simulink model "Battery_model_driving_cycle"  (R2019b)
settings: Solver=VariableStepAuto  StartTime=0.0  StopTime=10  RelTol=1e-3
undefined symbols (not defined in the file): A_frontal, air_density, Cn, Crate, Crate_fast, Cth, cv, fv, g, Gair, Gliquid, kt, m, Ob, Pn, Q_init, Rs1, rw, SOC_in, Temperature_BP, Tn, Vn
libraries: powerlib x27, simulink x10, drivingcycle_lib x2, powerlib_meascontrol x1
settings Model: Creator=Checco  LastModifiedBy=secch
settings SolverCC: ZeroCrossAlgorithm=Adaptive
settings DebuggingCC: IgnoredZcDiagnostic=none  ArithmeticOperatorsInVariantConditions=warning
settings SFSimCC: CustomCodeUndefinedFunction=UseInterfaceOnly

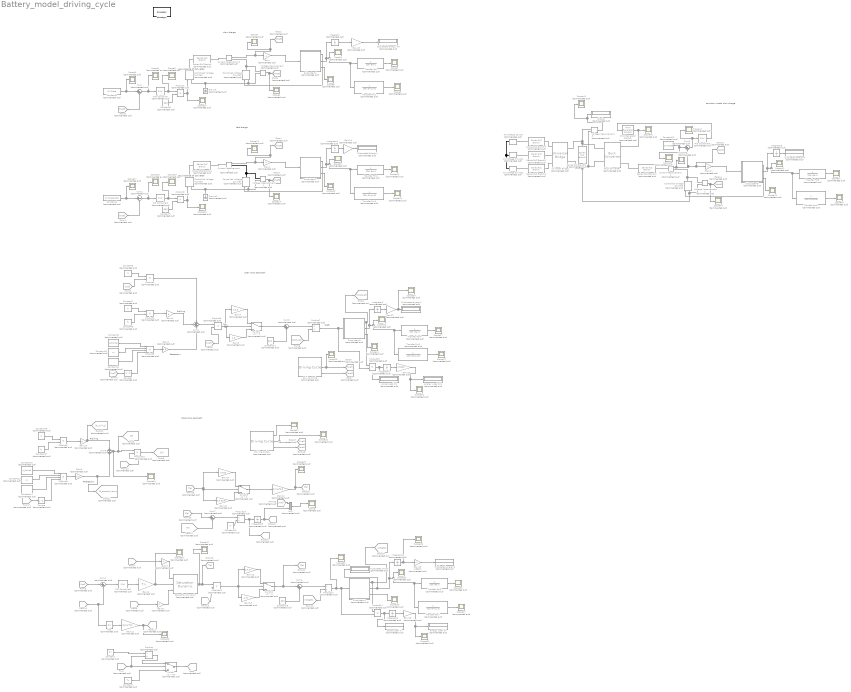
== system Battery_model_driving_cycle ==
  note: slow charge
  note: fast charge
  note: close loop approach
  note: open loop approach
  note: Ibatt
  note: Pm _
  note: Rrolling
  note: Raereodyn
  note: equivalence of converter
  note: equivalence of converter
  note: Rrolling
  note: Raereodyn
  note: complex model slow charge
  AC Voltage Source : powerlib/Electrical Sources/AC Voltage Source  Commented=on  Amplitude=230*sqrt(3)  Phase=0  Frequency=50  SampleTime=0  Measurements=None  BusType=swing  Pref=10e3  Qref=0  Qmin=-inf  Qmax=+inf
      settings: SourceProductName=Simscape Electrical
  AC Voltage Source1 : powerlib/Electrical Sources/AC Voltage Source  Commented=on  Amplitude=230*sqrt(3)  Phase=-120  Frequency=50  SampleTime=0  Measurements=None  BusType=swing  Pref=10e3  Qref=0  Qmin=-inf  Qmax=+inf
      settings: SourceProductName=Simscape Electrical
  AC Voltage Source2 : powerlib/Electrical Sources/AC Voltage Source  Commented=on  Amplitude=230*sqrt(3)  Phase=-240  Frequency=50  SampleTime=0  Measurements=None  BusType=swing  Pref=10e3  Qref=0  Qmin=-inf  Qmax=+inf
      settings: SourceProductName=Simscape Electrical
  Abs : Abs  Commented=on
  Buck Converter : powerlib/Power Electronics/Buck Converter  Commented=on  ModelType=Switching devices  Ron=1e-3  Rs=1e6  Cs=inf  Vforward=[0,0]  Ron_Diode=1e-3  Rs_Diode=1e6  Cs_Diode=inf  Vf_Diode=1e-3  Rs_CurrentSource=inf
      settings: SourceProductName=Simscape Electrical  SourceProductBaseCode=PS
  Constant : Constant  Commented=on  Value=Pn
  Constant1 : Constant  Commented=on  Value=Tn
  Constant10 : Constant  Commented=on  Value=cv
  Constant11 : Constant  Commented=on  Value=air_density
  Constant12 : Constant  Commented=on  Value=800
  Constant13 : Constant  Commented=on  Value=cv
  Constant14 : Constant  Commented=on  Value=air_density
  Constant{6..7,15,19} (4 alike) : Constant  Commented=on  Value=m
  Constant16 : Constant  Commented=on  Value=A_frontal
  Constant17 : Constant  Commented=on  Value=fv
  Constant18 : Constant  Commented=on  Value=800
  Constant2 : Constant  Commented=on  Value=Cn*Crate  SampleTime=-1
  Constant20 : Constant  Commented=on  Value=Cn*Crate  SampleTime=-1
  Constant3 : Constant  Commented=on  Value=560
  Constant4 : Constant  Commented=on  Value=Cn*Crate_fast  SampleTime=-1
  Constant5 : Constant  Commented=on  Value=560
  Constant8 : Constant  Commented=on  Value=A_frontal
  Constant9 : Constant  Commented=on  Value=fv
  Controlled Voltage Source1 : powerlib/Electrical Sources/Controlled Voltage Source  Commented=on  Initialize=off  Source_Type=DC  Amplitude=0.2*Cn  Phase=0  Frequency=0  Measurements=None
      settings: SourceProductName=Simscape Electrical
  Controlled Voltage Source2 : powerlib/Electrical Sources/Controlled Voltage Source  Commented=on  Initialize=off  Source_Type=DC  Amplitude=0  Phase=0  Frequency=0  Measurements=None
      settings: SourceProductName=Simscape Electrical
  Controlled Voltage Source3 : powerlib/Electrical Sources/Controlled Voltage Source  Commented=on  Initialize=off  Source_Type=DC  Amplitude=0.2*Cn  Phase=0  Frequency=0  Measurements=None
      settings: SourceProductName=Simscape Electrical
  Controlled Voltage Source4 : powerlib/Electrical Sources/Controlled Voltage Source  Commented=on  Initialize=off  Source_Type=DC  Amplitude=0  Phase=0  Frequency=0  Measurements=None
      settings: SourceProductName=Simscape Electrical
  Controlled Voltage Source6 : powerlib/Electrical Sources/Controlled Voltage Source  Commented=on  Initialize=off  Source_Type=DC  Amplitude=0  Phase=0  Frequency=0  Measurements=None
      settings: SourceProductName=Simscape Electrical
  Current Measurement : powerlib/Measurements/Current Measurement  Commented=on  PhasorSimulation=off  OutputType=Complex  PSBequivalent=0
      settings: SourceProductName=Simscape Electrical
  Current Measurement1 : powerlib/Measurements/Current Measurement  Commented=on  PhasorSimulation=off  OutputType=Complex  PSBequivalent=0
      settings: SourceProductName=Simscape Electrical
  Current Measurement2 : powerlib/Measurements/Current Measurement  Commented=on  PhasorSimulation=off  OutputType=Complex  PSBequivalent=0
      settings: SourceProductName=Simscape Electrical
  Display : Display  Commented=on
  Dissipated energy Wh : Display  Commented=on
  Dissipated energy{1..4} (4 alike) : Display  Commented=on
  Dissipated power : Display  Commented=on
  Driving Cycle : drivingcycle_lib/Driving Cycle  Commented=on  CycleName=NEDC  CycleRepeatsForever=off
      settings: SourceProductName=Driving Cycle Blockset
  Driving Cycle1 : drivingcycle_lib/Driving Cycle  Commented=on  CycleName=NEDC  CycleRepeatsForever=off
      settings: SourceProductName=Driving Cycle Blockset
  From : From  Commented=on  GotoTag=Omega
  From1 : From  Commented=on  GotoTag=Ibatt
  From10 : From  Commented=on  GotoTag=Vmeas
  From11 : From  Commented=on  GotoTag=Vmeas
  From12 : From  Commented=on  GotoTag=Vmeas
  From13 : From  Commented=on  GotoTag=Omega
  From14 : From  Commented=on  GotoTag=Vbatt
  From15 : From  Commented=on  GotoTag=Te
  From16 : From  Commented=on  GotoTag=Fe
  From17 : From  Commented=on  GotoTag=Fr
  From{4..5,9,18} (4 alike) : From  Commented=on  GotoTag=Vref
  From2 : From  Commented=on  GotoTag=Ibatt
  From3 : From  Commented=on  GotoTag=aref
  From6 : From  Commented=on  GotoTag=Vbatt_ref
  From7 : From  Commented=on  GotoTag=Tmax
  From8 : From  Commented=on  GotoTag=Tmax
  Gain{,1,8,17} (4 alike) : Gain  Commented=on  Gain=-1
  Gain10 : Gain  Commented=on  Gain=g
  Gain11 : Gain  Commented=on  Gain=1/rw*kt
  Gain12 : Gain  Commented=on  Gain=1/0.97
  Gain13 : Gain  Commented=on  Gain=0.97
  Gain14 : Gain  Commented=on  Gain=0.825
  Gain15 : Gain  Commented=on  Gain=1/0.825
  Gain16 : Gain  Commented=on  Gain=1/rw*kt
  Gain{18..23} (6 alike) : Gain  Commented=on  Gain=1/3600
  Gain2 : Gain  Commented=on  Gain=0.5
  Gain3 : Gain  Commented=on  Gain=g
  Gain4 : Gain  Commented=on  Gain=1/0.8
  Gain5 : Gain  Commented=on  Gain=0.8
  Gain6 : Gain  Commented=on  Gain=Tn
  Gain7 : Gain  Commented=on
  Gain9 : Gain  Commented=on  Gain=0.5
  Goto : Goto  Commented=on  GotoTag=Tmax
  Goto{1,3,14,19} (4 alike) : Goto  Commented=on  GotoTag=Vbatt
  Goto10 : Goto  Commented=on  GotoTag=R_rolling
  Goto11 : Goto  Commented=on  GotoTag=R_aereodynamic
  Goto12 : Goto  Commented=on  GotoTag=Omega
  Goto13 : Goto  Commented=on  GotoTag=Te
  Goto15 : Goto  Commented=on  GotoTag=Fe
  Goto16 : Goto  Commented=on  GotoTag=Vmeas
  Goto17 : Goto  Commented=on  GotoTag=Vref
  Goto18 : Goto  Commented=on  GotoTag=aref
  Goto2 : Goto  Commented=on  GotoTag=Ibatt
  Goto20 : Goto  Commented=on  GotoTag=ameas
  Goto21 : Goto  Commented=on  GotoTag=Pe
  Goto22 : Goto  Commented=on  GotoTag=Ibatt
  Goto4 : Goto  Commented=on  GotoTag=Ibatt
  Goto5 : Goto  Commented=on  GotoTag=Vbatt_ref
  Goto6 : Goto  Commented=on  GotoTag=Vref
  Goto7 : Goto  Commented=on  GotoTag=aref
  Goto8 : Goto  Commented=on  GotoTag=Fr
  Goto9 : Goto  Commented=on  GotoTag=Pr
  Ground : powerlib/Elements/Ground  Commented=on  LConnTagsString=a
      settings: SourceProductName=Simscape Electrical
  Ground1 : powerlib/Elements/Ground  Commented=on  LConnTagsString=a
      settings: SourceProductName=Simscape Electrical
  Integrator{,1..7} (8 alike) : Integrator  Commented=on
  Mux : Mux  Commented=on  Inputs=2
  PID Controller : simulink/Continuous/PID Controller  Commented=on  Controller=PI  Form=Parallel  TimeDomain=Continuous-time  SampleTime=-1  IntegratorMethod=Forward Euler  FilterMethod=Forward Euler  ControllerParametersSource=internal  P=0.01  I=1  D=0  UseFilter=on  N=100  TunerSelectOption=Transfer Function Based (PID Tuner App)  InitialConditionSource=internal  InitialConditionForIntegrator=370/560  InitialConditionForFilter=0  DifferentiatorICPrevScaledInput=0  ExternalReset=none  TrackingMode=off  Kt=1  LimitOutput=on  UpperSaturationLimit=1  LowerSaturationLimit=0  LinearizeAsGain=on  AntiWindupMode=none  Kb=1  POutMin=[]  POutMax=[]  IOutMin=[]  IOutMax=[]  DOutMin=[]  DOutMax=[]  NOutMin=[]  NOutMax=[]  SumOutMin=[]  SumOutMax=[]  SaturationOutMin=[]  SaturationOutMax=[]  PParamMin=[]  PParamMax=[]  IParamMin=[]  IParamMax=[]  DParamMin=[]  DParamMax=[]  NParamMin=[]  NParamMax=[]  KbParamMin=[]  KbParamMax=[]  KtParamMin=[]  KtParamMax=[]  KbOutMin=[]  KbOutMax=[]  KtOutMin=[]  KtOutMax=[]  IntegratorOutMin=[]  IntegratorOutMax=[]  FilterOutMin=[]  FilterOutMax=[]  SumI1OutMin=[]  SumI1OutMax=[]  SumI2OutMin=[]  SumI2OutMax=[]  SumI3OutMin=[]  SumI3OutMax=[]  SumI4OutMin=[]  SumI4OutMax=[]  SumDOutMin=[]  SumDOutMax=[]  DifferentiatorOutMin=[]  DifferentiatorOutMax=[]  FilterDiffOutCoefMin=[]  FilterDiffOutCoefMax=[]  ReciprocalOutMin=[]  ReciprocalOutMax=[]  SumDenOutMin=[]  SumDenOutMax=[]  SumNumOutMin=[]  SumNumOutMax=[]  DivideOutMin=[]  DivideOutMax=[]  IntegratorContinuousStateAttributes=''  IntegratorStateMustResolveToSignalObject=off  IntegratorRTWStateStorageClass=Auto  FilterContinuousStateAttributes=''  FilterStateMustResolveToSignalObject=off  FilterRTWStateStorageClass=Auto  ParallelPVariant=InternalParameters  IdealPVariant=Disabled  IVariant=InternalParameters  DVariant=Disabled  IntegratorVariant=Continuous  SatVariant=Enabled  AWVariant=Passthrough  PCopyVariant=Disabled  TRVariant=Disabled  FdbkBlocksVariant=Forward  IdealPFdbkVariant=Disabled  SatFdbkVariant=Disabled  DerivativeFilterVariant=Disabled  NVariant=Disabled  NCopyVariant=Disabled_SignalSpec  FilterICVariant=Disabled  IntegratorICVariant=InternalICs  ExternalResetVariant=Disabled  TRSumVariant=Passthrough  SumFdbkVariant=Disabled  SumVariant=Sum_PI
  PID Controller1 : simulink/Continuous/PID Controller  Commented=on  Controller=PI  Form=Parallel  TimeDomain=Continuous-time  SampleTime=-1  IntegratorMethod=Forward Euler  FilterMethod=Forward Euler  ControllerParametersSource=internal  P=0.01  I=1  D=0  UseFilter=on  N=100  TunerSelectOption=Transfer Function Based (PID Tuner App)  InitialConditionSource=internal  InitialConditionForIntegrator=370/560  InitialConditionForFilter=0  DifferentiatorICPrevScaledInput=0  ExternalReset=none  TrackingMode=off  Kt=1  LimitOutput=on  UpperSaturationLimit=1  LowerSaturationLimit=0  LinearizeAsGain=on  AntiWindupMode=none  Kb=1  POutMin=[]  POutMax=[]  IOutMin=[]  IOutMax=[]  DOutMin=[]  DOutMax=[]  NOutMin=[]  NOutMax=[]  SumOutMin=[]  SumOutMax=[]  SaturationOutMin=[]  SaturationOutMax=[]  PParamMin=[]  PParamMax=[]  IParamMin=[]  IParamMax=[]  DParamMin=[]  DParamMax=[]  NParamMin=[]  NParamMax=[]  KbParamMin=[]  KbParamMax=[]  KtParamMin=[]  KtParamMax=[]  KbOutMin=[]  KbOutMax=[]  KtOutMin=[]  KtOutMax=[]  IntegratorOutMin=[]  IntegratorOutMax=[]  FilterOutMin=[]  FilterOutMax=[]  SumI1OutMin=[]  SumI1OutMax=[]  SumI2OutMin=[]  SumI2OutMax=[]  SumI3OutMin=[]  SumI3OutMax=[]  SumI4OutMin=[]  SumI4OutMax=[]  SumDOutMin=[]  SumDOutMax=[]  DifferentiatorOutMin=[]  DifferentiatorOutMax=[]  FilterDiffOutCoefMin=[]  FilterDiffOutCoefMax=[]  ReciprocalOutMin=[]  ReciprocalOutMax=[]  SumDenOutMin=[]  SumDenOutMax=[]  SumNumOutMin=[]  SumNumOutMax=[]  DivideOutMin=[]  DivideOutMax=[]  IntegratorContinuousStateAttributes=''  IntegratorStateMustResolveToSignalObject=off  IntegratorRTWStateStorageClass=Auto  FilterContinuousStateAttributes=''  FilterStateMustResolveToSignalObject=off  FilterRTWStateStorageClass=Auto  ParallelPVariant=InternalParameters  IdealPVariant=Disabled  IVariant=InternalParameters  DVariant=Disabled  IntegratorVariant=Continuous  SatVariant=Enabled  AWVariant=Passthrough  PCopyVariant=Disabled  TRVariant=Disabled  FdbkBlocksVariant=Forward  IdealPFdbkVariant=Disabled  SatFdbkVariant=Disabled  DerivativeFilterVariant=Disabled  NVariant=Disabled  NCopyVariant=Disabled_SignalSpec  FilterICVariant=Disabled  IntegratorICVariant=InternalICs  ExternalResetVariant=Disabled  TRSumVariant=Passthrough  SumFdbkVariant=Disabled  SumVariant=Sum_PI
  PID Controller2 : simulink/Continuous/PID Controller  Commented=on  Controller=PI  Form=Parallel  TimeDomain=Continuous-time  SampleTime=-1  IntegratorMethod=Forward Euler  FilterMethod=Forward Euler  ControllerParametersSource=internal  P=1  I=100  D=0  UseFilter=on  N=100  TunerSelectOption=Transfer Function Based (PID Tuner App)  InitialConditionSource=internal  InitialConditionForIntegrator=0  InitialConditionForFilter=0  DifferentiatorICPrevScaledInput=0  ExternalReset=none  TrackingMode=off  Kt=1  LimitOutput=on  UpperSaturationLimit=1  LowerSaturationLimit=-1  LinearizeAsGain=on  AntiWindupMode=none  Kb=1  POutMin=[]  POutMax=[]  IOutMin=[]  IOutMax=[]  DOutMin=[]  DOutMax=[]  NOutMin=[]  NOutMax=[]  SumOutMin=[]  SumOutMax=[]  SaturationOutMin=[]  SaturationOutMax=[]  PParamMin=[]  PParamMax=[]  IParamMin=[]  IParamMax=[]  DParamMin=[]  DParamMax=[]  NParamMin=[]  NParamMax=[]  KbParamMin=[]  KbParamMax=[]  KtParamMin=[]  KtParamMax=[]  KbOutMin=[]  KbOutMax=[]  KtOutMin=[]  KtOutMax=[]  IntegratorOutMin=[]  IntegratorOutMax=[]  FilterOutMin=[]  FilterOutMax=[]  SumI1OutMin=[]  SumI1OutMax=[]  SumI2OutMin=[]  SumI2OutMax=[]  SumI3OutMin=[]  SumI3OutMax=[]  SumI4OutMin=[]  SumI4OutMax=[]  SumDOutMin=[]  SumDOutMax=[]  DifferentiatorOutMin=[]  DifferentiatorOutMax=[]  FilterDiffOutCoefMin=[]  FilterDiffOutCoefMax=[]  ReciprocalOutMin=[]  ReciprocalOutMax=[]  SumDenOutMin=[]  SumDenOutMax=[]  SumNumOutMin=[]  SumNumOutMax=[]  DivideOutMin=[]  DivideOutMax=[]  IntegratorContinuousStateAttributes=''  IntegratorStateMustResolveToSignalObject=off  IntegratorRTWStateStorageClass=Auto  FilterContinuousStateAttributes=''  FilterStateMustResolveToSignalObject=off  FilterRTWStateStorageClass=Auto  ParallelPVariant=InternalParameters  IdealPVariant=Disabled  IVariant=InternalParameters  DVariant=Disabled  IntegratorVariant=Continuous  SatVariant=Enabled  AWVariant=Passthrough  PCopyVariant=Disabled  TRVariant=Disabled  FdbkBlocksVariant=Forward  IdealPFdbkVariant=Disabled  SatFdbkVariant=Disabled  DerivativeFilterVariant=Disabled  NVariant=Disabled  NCopyVariant=Disabled_SignalSpec  FilterICVariant=Disabled  IntegratorICVariant=InternalICs  ExternalResetVariant=Disabled  TRSumVariant=Passthrough  SumFdbkVariant=Disabled  SumVariant=Sum_PI
  PID Controller3 : simulink/Continuous/PID Controller  Commented=on  Controller=PI  Form=Parallel  TimeDomain=Continuous-time  SampleTime=-1  IntegratorMethod=Forward Euler  FilterMethod=Forward Euler  ControllerParametersSource=internal  P=0.01  I=1  D=0  UseFilter=on  N=100  TunerSelectOption=Transfer Function Based (PID Tuner App)  InitialConditionSource=internal  InitialConditionForIntegrator=Vn/560  InitialConditionForFilter=0  DifferentiatorICPrevScaledInput=0  ExternalReset=none  TrackingMode=off  Kt=1  LimitOutput=on  UpperSaturationLimit=1  LowerSaturationLimit=0  LinearizeAsGain=on  AntiWindupMode=none  Kb=1  POutMin=[]  POutMax=[]  IOutMin=[]  IOutMax=[]  DOutMin=[]  DOutMax=[]  NOutMin=[]  NOutMax=[]  SumOutMin=[]  SumOutMax=[]  SaturationOutMin=[]  SaturationOutMax=[]  PParamMin=[]  PParamMax=[]  IParamMin=[]  IParamMax=[]  DParamMin=[]  DParamMax=[]  NParamMin=[]  NParamMax=[]  KbParamMin=[]  KbParamMax=[]  KtParamMin=[]  KtParamMax=[]  KbOutMin=[]  KbOutMax=[]  KtOutMin=[]  KtOutMax=[]  IntegratorOutMin=[]  IntegratorOutMax=[]  FilterOutMin=[]  FilterOutMax=[]  SumI1OutMin=[]  SumI1OutMax=[]  SumI2OutMin=[]  SumI2OutMax=[]  SumI3OutMin=[]  SumI3OutMax=[]  SumI4OutMin=[]  SumI4OutMax=[]  SumDOutMin=[]  SumDOutMax=[]  DifferentiatorOutMin=[]  DifferentiatorOutMax=[]  FilterDiffOutCoefMin=[]  FilterDiffOutCoefMax=[]  ReciprocalOutMin=[]  ReciprocalOutMax=[]  SumDenOutMin=[]  SumDenOutMax=[]  SumNumOutMin=[]  SumNumOutMax=[]  DivideOutMin=[]  DivideOutMax=[]  IntegratorContinuousStateAttributes=''  IntegratorStateMustResolveToSignalObject=off  IntegratorRTWStateStorageClass=Auto  FilterContinuousStateAttributes=''  FilterStateMustResolveToSignalObject=off  FilterRTWStateStorageClass=Auto  ParallelPVariant=InternalParameters  IdealPVariant=Disabled  IVariant=InternalParameters  DVariant=Disabled  IntegratorVariant=Continuous  SatVariant=Enabled  AWVariant=Passthrough  PCopyVariant=Disabled  TRVariant=Disabled  FdbkBlocksVariant=Forward  IdealPFdbkVariant=Disabled  SatFdbkVariant=Disabled  DerivativeFilterVariant=Disabled  NVariant=Disabled  NCopyVariant=Disabled_SignalSpec  FilterICVariant=Disabled  IntegratorICVariant=InternalICs  ExternalResetVariant=Disabled  TRSumVariant=Passthrough  SumFdbkVariant=Disabled  SumVariant=Sum_PI
  PWM Generator (DC-DC) : powerlib_meascontrol/Pulse & Signal Generators/PWM Generator (DC-DC)  Commented=on  Fsw=5000  Ts=0
      settings: SourceProductName=Simscape Electrical
  Product{,7,12..13} (4 alike) : Product  Commented=on  Inputs=*/
  Product{1..4,6,8,10..11} (8 alike) : Product  Commented=on
  Product14 : Product  Commented=on  Inputs=**
  Product15 : Product  Commented=on  Inputs=**
  Product5 : Product  Commented=on  Inputs=4
  Product9 : Product  Commented=on  Inputs=4
  Saturation Dynamic : simulink/Discontinuities/Saturation Dynamic  Commented=on  OutMin=[]  OutMax=[]  OutDataTypeStr=Inherit: Same as second input  OutDataType=fixdt(1, 16)  OutScaling=2^-10  DoSatur=off
  Scope{,1..51} (52 alike) : Scope  Commented=on
  Series RLC Branch : powerlib/Elements/Series RLC Branch  Commented=on  LConnTagsString=__new0  RConnTagsString=__new0  BranchType=RL  Resistance=0.0001  Inductance=0.01  SetiL0=off  InitialCurrent=0  Capacitance=1e-6  Setx0=off  InitialVoltage=0  Measurements=None
      settings: SourceProductName=Simscape Electrical
  Series RLC Branch1 : powerlib/Elements/Series RLC Branch  Commented=on  LConnTagsString=__new0  RConnTagsString=__new0  BranchType=RL  Resistance=0.0001  Inductance=0.01  SetiL0=off  InitialCurrent=0  Capacitance=1e-6  Setx0=off  InitialVoltage=0  Measurements=None
      settings: SourceProductName=Simscape Electrical
  Series RLC Branch2 : powerlib/Elements/Series RLC Branch  Commented=on  LConnTagsString=__new0  RConnTagsString=__new0  BranchType=RL  Resistance=3  Inductance=1e-3  SetiL0=off  InitialCurrent=0  Capacitance=1e-6  Setx0=off  InitialVoltage=0  Measurements=None
      settings: SourceProductName=Simscape Electrical
  Series RLC Branch3 : powerlib/Elements/Series RLC Branch  Commented=on  LConnTagsString=__new0  RConnTagsString=__new0  BranchType=RL  Resistance=3  Inductance=1e-3  SetiL0=off  InitialCurrent=0  Capacitance=1e-6  Setx0=off  InitialVoltage=0  Measurements=None
      settings: SourceProductName=Simscape Electrical
  Series RLC Branch4 : powerlib/Elements/Series RLC Branch  Commented=on  LConnTagsString=__new0  RConnTagsString=__new0  BranchType=RL  Resistance=3  Inductance=1e-3  SetiL0=off  InitialCurrent=0  Capacitance=1e-6  Setx0=off  InitialVoltage=0  Measurements=None
      settings: SourceProductName=Simscape Electrical
  Series RLC Branch6 : powerlib/Elements/Series RLC Branch  Commented=on  LConnTagsString=__new0  RConnTagsString=__new0  BranchType=C  Resistance=0.0001  Inductance=0.01  SetiL0=off  InitialCurrent=0  Capacitance=600e-6  Setx0=off  InitialVoltage=0  Measurements=None
      settings: SourceProductName=Simscape Electrical
  Series RLC Branch7 : powerlib/Elements/Series RLC Branch  Commented=on  LConnTagsString=__new0  RConnTagsString=__new0  BranchType=RL  Resistance=0.0001  Inductance=0.01  SetiL0=off  InitialCurrent=0  Capacitance=1e-6  Setx0=off  InitialVoltage=0  Measurements=None
      settings: SourceProductName=Simscape Electrical
  Square : Math  Commented=on  Operator=square  SignedPower=off  SaturateOnIntegerOverflow=on
  Square1 : Math  Commented=on  Operator=square  SignedPower=off  SaturateOnIntegerOverflow=on
  Subsystem1 : Subsystem  Commented=on  mask{Em=|, R0=0.0036, SOC_BP=|, BattCap=31, SOC_ini=20, Ns=100, Np=3}
      mask Em=|
      | [3;
      | 3.5 ;
      | 3.67 ;
      | 3.7 ;
      | 3.71 ;
      | 3.72 ;
      | 3.73 ;
      | 3.74 ;
      | 3.75 ;
      | 3.84;
      | 4.2]
      mask SOC_BP=|
      | [0
      | 0.1
      | 0.2
      | 0.3
      | 0.4
      | 0.5
      | 0.6
      | 0.7
      | 0.8
      | 0.9
      | 1]
      mask prompts: Em "Open circuit voltage table data, Em [V]:"; R0 "Series resistance R0 [Ohm]:"; SOC_BP "State of charge breakpoints, SOC_BP []"; BattCap "Battery capacity, BattCap [Ah]"; SOC_ini "SOC ini [%]"; Ns "Num Series"; Np "Num Parallel"
      mask DialogControl Control3 Prompt: Single Module Data
      mask DialogControl Control2 Prompt: Connections
  Subsystem2 : Subsystem  Commented=on  mask{Em=|, R0=0.0036, SOC_BP=|, BattCap=31, SOC_ini=20, Ns=100, Np=3}
      mask Em=|
      | [3;
      | 3.5 ;
      | 3.67 ;
      | 3.7 ;
      | 3.71 ;
      | 3.72 ;
      | 3.73 ;
      | 3.74 ;
      | 3.75 ;
      | 3.84;
      | 4.2]
      mask SOC_BP=|
      | [0
      | 0.1
      | 0.2
      | 0.3
      | 0.4
      | 0.5
      | 0.6
      | 0.7
      | 0.8
      | 0.9
      | 1]
      mask prompts: Em "Open circuit voltage table data, Em [V]:"; R0 "Series resistance R0 [Ohm]:"; SOC_BP "State of charge breakpoints, SOC_BP []"; BattCap "Battery capacity, BattCap [Ah]"; SOC_ini "SOC ini [%]"; Ns "Num Series"; Np "Num Parallel"
      mask DialogControl Control3 Prompt: Single Module Data
      mask DialogControl Control2 Prompt: Connections
  Subsystem3 : Subsystem  Commented=on  mask{Em=|, R0=0.0036, SOC_BP=|, BattCap=31, SOC_ini=100, Ns=100, Np=3}
      mask Em=|
      | [3;
      | 3.5 ;
      | 3.67 ;
      | 3.7 ;
      | 3.71 ;
      | 3.72 ;
      | 3.73 ;
      | 3.74 ;
      | 3.75 ;
      | 3.84;
      | 4.2]
      mask SOC_BP=|
      | [0
      | 0.1
      | 0.2
      | 0.3
      | 0.4
      | 0.5
      | 0.6
      | 0.7
      | 0.8
      | 0.9
      | 1]
      mask prompts: Em "Open circuit voltage table data, Em [V]:"; R0 "Series resistance R0 [Ohm]:"; SOC_BP "State of charge breakpoints, SOC_BP []"; BattCap "Battery capacity, BattCap [Ah]"; SOC_ini "SOC ini [%]"; Ns "Num Series"; Np "Num Parallel"
      mask DialogControl Control3 Prompt: Single Module Data
      mask DialogControl Control2 Prompt: Connections
  Subsystem4 : Subsystem  Commented=on  mask{Em=|, R0=0.0036, SOC_BP=|, BattCap=31, SOC_ini=100, Ns=100, Np=3}
      mask Em=|
      | [3;
      | 3.5 ;
      | 3.67 ;
      | 3.7 ;
      | 3.71 ;
      | 3.72 ;
      | 3.73 ;
      | 3.74 ;
      | 3.75 ;
      | 3.84;
      | 4.2]
      mask SOC_BP=|
      | [0
      | 0.1
      | 0.2
      | 0.3
      | 0.4
      | 0.5
      | 0.6
      | 0.7
      | 0.8
      | 0.9
      | 1]
      mask prompts: Em "Open circuit voltage table data, Em [V]:"; R0 "Series resistance R0 [Ohm]:"; SOC_BP "State of charge breakpoints, SOC_BP []"; BattCap "Battery capacity, BattCap [Ah]"; SOC_ini "SOC ini [%]"; Ns "Num Series"; Np "Num Parallel"
      mask DialogControl Control3 Prompt: Single Module Data
      mask DialogControl Control2 Prompt: Connections
  Subsystem5 : Subsystem  Commented=on  mask{Em=|, R0=0.0036, SOC_BP=|, BattCap=31, SOC_ini=20, Ns=100, Np=3}
      mask Em=|
      | [3;
      | 3.5 ;
      | 3.67 ;
      | 3.7 ;
      | 3.71 ;
      | 3.72 ;
      | 3.73 ;
      | 3.74 ;
      | 3.75 ;
      | 3.84;
      | 4.2]
      mask SOC_BP=|
      | [0
      | 0.1
      | 0.2
      | 0.3
      | 0.4
      | 0.5
      | 0.6
      | 0.7
      | 0.8
      | 0.9
      | 1]
      mask prompts: Em "Open circuit voltage table data, Em [V]:"; R0 "Series resistance R0 [Ohm]:"; SOC_BP "State of charge breakpoints, SOC_BP []"; BattCap "Battery capacity, BattCap [Ah]"; SOC_ini "SOC ini [%]"; Ns "Num Series"; Np "Num Parallel"
      mask DialogControl Control3 Prompt: Single Module Data
      mask DialogControl Control2 Prompt: Connections
  Sum{,1,4,7..8} (5 alike) : Sum  Commented=on  Inputs=|+-
  Sum2 : Sum  Commented=on  Inputs=+++
  Sum3 : Sum  Commented=on  Inputs=|++
  Sum5 : Sum  Commented=on
  Sum6 : Sum  Commented=on  Inputs=|++
  Switch : Switch  Commented=on  Criteria=u2 > Threshold  Threshold=Ob
  Switch1 : Switch  Commented=on  Criteria=u2 > Threshold
  Switch2 : Switch  Commented=on  Criteria=u2 > Threshold
  Switch3 : Switch  Commented=on  Criteria=u2 > Threshold
  Transfer Fcn{,2,4,6,8} (5 alike) : TransferFcn  Commented=on  Denominator=[Cth Gair]
  Transfer Fcn{1,3,5,7,9} (5 alike) : TransferFcn  Commented=on  Denominator=[Cth Gliquid]
  Universal Bridge : powerlib/Power Electronics/Universal Bridge  Commented=on  Arms=3  SnubberResistance=1e5  SnubberCapacitance=inf  Device=Diodes  Ron=1e-3  Lon=0  ForwardVoltages="[  0  0  ]"  ForwardVoltage=0  GTOparameters=[ 10e-6 , 20e-6 ]  IGBTparameters=[ 1e-6 , 2e-6 ]  Measurements=None  Measurements_2=None  converterType=Rectifier
      settings: SourceProductName=Simscape Electrical
  Voltage Measurement{,1..3} (4 alike) : powerlib/Measurements/Voltage Measurement  Commented=on  PhasorSimulation=off  OutputType=Complex  PSBequivalent=0
      settings: SourceProductName=Simscape Electrical
  energy used wh : Display  Commented=on
  energy used wh1 : Display  Commented=on
  power used W : Display  Commented=on
  power used W1 : Display  Commented=on
  powergui : powerlib/powergui  Priority=1  SimulationMode=Continuous  SampleTime=50e-6  frequency=60  Iterations=50  frequencyindice=0  Pbase=100e6  ErrMax=1e-4  UnitsV=kV  UnitsW=MW  buscounter=0  FunctionMessages=off  echomessages=off  EnableUseOfTLC=off  CurrentSourceSwitches=off  DisableSnubberDevices=off  DisableRonSwitches=off  DisableVfSwitches=off  DisplayEquations=off  AutomaticDiscreteSolvers=off  SolverType=Tustin/Backward Euler (TBE)  Interpol=off  ExternalGateDelay=off  methode=off  Ts=100  x0status=blocks  SPID=on  SwTol=0  HookPort=off  NonlinearTolerance=1e-4  nMaxIteration=100  ContinueOnMaxIteration=off  RestoreLinks=warning  ResistiveCurrentMeasurement=off  Frange=[0:2:500]  Ylog=off  Xlog=on  ShowGrid=off  save=off  variable=ZData  structure=0  ZoomFFT=off  StartTime=0.0  cycles=1  DisplayStyle=1  fundamental=60  FreqAxis=off  MaxFrequency=1000  frequencyindicesteady=1  RmsSteady=1  display=off
      settings: SourceProductName=Simscape Electrical
  wires:
  From2/1 -> Sum/2
  Sum/1 -> Scope5/1, PID Controller/1
  PID Controller/1 -> Scope8/1, Product1/1
  Constant3/1 -> Product1/2
  Product1/1 -> Scope10/1, Controlled Voltage Source1/1
  Voltage Measurement/1 -> Scope4/1, Goto1/1
  Current Measurement/1 -> Goto2/1, Scope7/1, Gain/1
  Gain/1 -> Subsystem1/1(Ibatt)
  Subsystem1/2(Ploss) -> Scope1/1, Transfer Fcn1/1, Transfer Fcn/1, Integrator/1
  Integrator/1 -> Gain20/1
  Subsystem1/3(SOC) -> Scope9/1
  Transfer Fcn/1 -> Scope2/1
  Transfer Fcn1/1 -> Scope3/1
  Subsystem1/1(Vbatt) -> Controlled Voltage Source2/1
  Constant2/1 -> Scope6/1, Sum/1
  Constant4/1 -> Sum1/1, Scope17/1
  Subsystem2/1(Vbatt) -> Controlled Voltage Source4/1
  Transfer Fcn3/1 -> Scope14/1
  Transfer Fcn2/1 -> Scope13/1
  Subsystem2/3(SOC) -> Scope20/1
  Integrator1/1 -> Gain21/1
  Subsystem2/2(Ploss) -> Integrator1/1, Transfer Fcn2/1, Transfer Fcn3/1, Scope11/1
  Gain1/1 -> Subsystem2/1(Ibatt)
  Current Measurement1/1 -> Gain1/1, Scope18/1, Goto4/1
  Voltage Measurement1/1 -> Goto3/1, Scope15/1
  Product2/1 -> Controlled Voltage Source3/1, Scope12/1
  Constant5/1 -> Product2/2
  PID Controller1/1 -> Product2/1, Scope19/1
  Sum1/1 -> PID Controller1/1, Scope16/1
  From1/1 -> Sum1/2
  Constant6/1 -> Product3/1
  From3/1 -> Product3/2
  Constant9/1 -> Product4/2
  Constant7/1 -> Product4/1
  Constant8/1 -> Product5/1
  Constant10/1 -> Product5/2
  Constant11/1 -> Product5/3
  From4/1 -> Square1/1
  Product5/1 -> Gain2/1
  Product4/1 -> Gain3/1
  Product3/1 -> Sum2/1
  Gain3/1 -> Sum2/2
  Gain2/1 -> Sum2/3
  Sum2/1 -> Product6/1
  From5/1 -> Product6/2
  Product6/1 -> Gain4/1, Gain5/1, Switch1/2
  Gain5/1 -> Switch1/3
  Gain4/1 -> Switch1/1
  Switch1/1 -> Sum3/1
  Constant12/1 -> Sum3/2
  Sum3/1 -> Product7/1
  From6/1 -> Product7/2
  Subsystem3/2(Ploss) -> Integrator2/1, Scope21/1, Transfer Fcn5/1, Transfer Fcn4/1
  Subsystem3/3(SOC) -> Scope24/1
  Transfer Fcn4/1 -> Scope22/1
  Transfer Fcn5/1 -> Scope23/1
  Product7/1 -> Product15/2, Subsystem3/1(Ibatt)
  Integrator2/1 -> Gain22/1
  Subsystem3/1(Vbatt) -> Goto5/1, Product15/1
  PID Controller2/1 -> Gain6/1
  Gain6/1 -> Scope33/1, Saturation Dynamic/2
  Gain8/1 -> Saturation Dynamic/3
  Gain7/1 -> Saturation Dynamic/1
  From7/1 -> Gain7/1
  From8/1 -> Gain8/1
  From9/1 -> Sum4/1
  Sum4/1 -> PID Controller2/1
  From10/1 -> Abs/1, Sum4/2
  Driving Cycle/2 -> Scope29/1, Goto6/1
  Driving Cycle/3 -> Goto7/1
  Product9/1 -> Gain9/1
  Constant14/1 -> Product9/3
  Gain9/1 -> Sum5/2, Goto11/1
  Constant16/1 -> Product9/1
  From11/1 -> Square/1
  Constant13/1 -> Product9/2
  Gain10/1 -> Sum5/1, Goto10/1
  Constant15/1 -> Product8/1
  Constant17/1 -> Product8/2
  Product8/1 -> Gain10/1
  Sum5/1 -> Scope34/1, Goto8/1, Product10/1
  From12/1 -> Product10/2
  Product10/1 -> Goto9/1
  Abs/1 -> Gain11/1
  Gain11/1 -> Scope39/1, Goto12/1
  Saturation Dynamic/1 -> Scope32/1, Goto13/1, Product11/1
  From13/1 -> Product11/2
  Product11/1 -> Gain12/1, Gain13/1, Switch2/2
  Constant18/1 -> Sum6/2
  Switch2/1 -> Goto21/1, Sum6/1
  Sum6/1 -> Product12/1
  From14/1 -> Product12/2
  Gain12/1 -> Switch2/1
  Gain13/1 -> Switch2/3
  Product/1 -> Switch/1
  Constant1/1 -> Switch/3
  Constant/1 -> Product/1
  From/1 -> Product/2, Switch/2
  Switch/1 -> Goto/1
  Gain15/1 -> Switch3/3
  Gain14/1 -> Switch3/1
  From15/1 -> Switch3/2, Gain15/1, Gain14/1
  Switch3/1 -> Gain16/1
  Gain16/1 -> Scope35/1, Goto15/1
  From16/1 -> Sum7/1
  From17/1 -> Sum7/2
  Sum7/1 -> Product13/1
  Constant19/1 -> Product13/2
  Product13/1 -> Goto20/1, Integrator3/1
  Integrator3/1 -> Mux/2, Goto16/1
  Driving Cycle1/3 -> Goto18/1
  Driving Cycle1/2 -> Scope31/1, Goto17/1
  Product12/1 -> Scope38/1, Product14/2, Subsystem4/1(Ibatt)
  Subsystem4/1(Vbatt) -> Product14/1, Goto19/1
  Integrator4/1 -> Scope36/1, Gain19/1
  Transfer Fcn7/1 -> Scope27/1
  Transfer Fcn6/1 -> Scope26/1
  Subsystem4/3(SOC) -> Scope28/1
  Subsystem4/2(Ploss) -> Dissipated power/1, Transfer Fcn6/1, Transfer Fcn7/1, Scope25/1, Integrator4/1
  Mux/1 -> Scope/1
  From18/1 -> Mux/1
  Driving Cycle1/1 -> Scope37/1
  Subsystem5/2(Ploss) -> Scope40/1, Transfer Fcn9/1, Transfer Fcn8/1, Integrator5/1
  Transfer Fcn9/1 -> Scope43/1
  Subsystem5/3(SOC) -> Scope49/1
  Gain17/1 -> Subsystem5/1(Ibatt)
  Current Measurement2/1 -> Scope45/1, Goto22/1, Gain17/1, Sum8/2
  Subsystem5/1(Vbatt) -> Controlled Voltage Source6/1
  Voltage Measurement2/1 -> Scope44/1, Goto14/1
  Transfer Fcn8/1 -> Scope42/1
  Integrator5/1 -> Dissipated energy4/1
  Constant20/1 -> Scope48/1, Sum8/1
  Sum8/1 -> Scope47/1, PID Controller3/1
  PID Controller3/1 -> PWM Generator (DC-DC)/1
  PWM Generator (DC-DC)/1 -> Buck Converter/1, Scope46/1
  Voltage Measurement3/1 -> Scope41/1, Display/1
  Product14/1 -> power used W/1, Integrator6/1
  Integrator6/1 -> Gain18/1
  Gain18/1 -> Scope50/1, energy used wh/1
  Gain19/1 -> Dissipated energy3/1
  Square/1 -> Product9/4
  Square1/1 -> Product5/4
  Gain20/1 -> Dissipated energy Wh/1
  Gain21/1 -> Dissipated energy1/1
  Gain22/1 -> Scope30/1, Dissipated energy2/1
  Gain23/1 -> energy used wh1/1, Scope51/1
  Integrator7/1 -> Gain23/1
  Product15/1 -> Integrator7/1, power used W1/1
  connections:
  Series RLC Branch/LConn1 -- Controlled Voltage Source1/RConn1
  Current Measurement/LConn1 -- Series RLC Branch/RConn1
  Controlled Voltage Source2/RConn1 -- Current Measurement/RConn1 -- Voltage Measurement/LConn1
  Controlled Voltage Source2/LConn1 -- Ground/LConn1 -- Controlled Voltage Source1/LConn1 -- Voltage Measurement/LConn2
  Current Measurement1/RConn1 -- Controlled Voltage Source4/RConn1 -- Voltage Measurement1/LConn1
  Voltage Measurement1/LConn2 -- Controlled Voltage Source4/LConn1 -- Controlled Voltage Source3/LConn1 -- Ground1/LConn1
  Current Measurement1/LConn1 -- Series RLC Branch1/RConn1
  Series RLC Branch1/LConn1 -- Controlled Voltage Source3/RConn1
  Voltage Measurement2/LConn1 -- Controlled Voltage Source6/RConn1 -- Current Measurement2/RConn1
  AC Voltage Source/RConn1 -- Series RLC Branch3/LConn1
  Series RLC Branch2/LConn1 -- AC Voltage Source1/RConn1
  Series RLC Branch4/LConn1 -- AC Voltage Source2/RConn1
  AC Voltage Source/LConn1 -- AC Voltage Source2/LConn1 -- AC Voltage Source1/LConn1
  Series RLC Branch2/RConn1 -- Universal Bridge/LConn2
  Universal Bridge/LConn1 -- Series RLC Branch3/RConn1
  Series RLC Branch4/RConn1 -- Universal Bridge/LConn3
  Series RLC Branch6/LConn1 -- Buck Converter/RConn1 -- Voltage Measurement3/LConn1 -- Universal Bridge/RConn1
  Series RLC Branch6/RConn1 -- Buck Converter/RConn2 -- Voltage Measurement3/LConn2 -- Voltage Measurement2/LConn2 -- Controlled Voltage Source6/LConn1 -- Universal Bridge/RConn2
  Series RLC Branch7/LConn1 -- Buck Converter/LConn1
  Current Measurement2/LConn1 -- Series RLC Branch7/RConn1

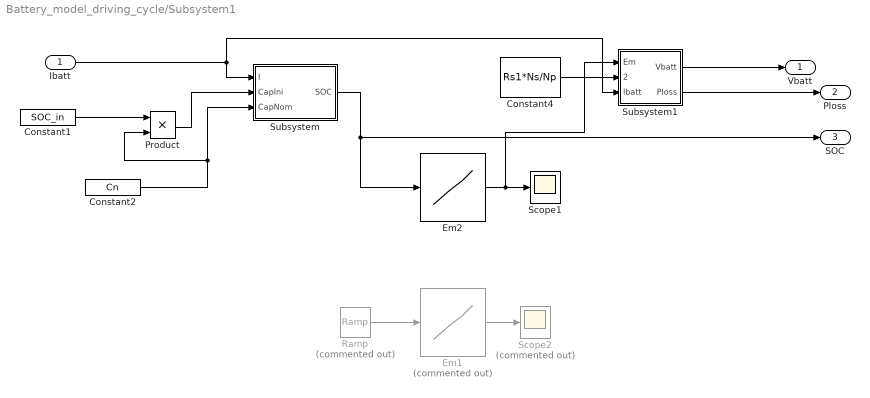
== system Battery_model_driving_cycle/Subsystem1 ==
  Ibatt : Inport
  Constant1 : Constant  Value=SOC_in  SampleTime=-1
  Constant2 : Constant  Value=Cn  SampleTime=-1
  Constant4 : Constant  Value=Rs1*Ns/Np  SampleTime=-1
  Em1 : Lookup_n-D  Commented=on  NumberOfTableDimensions=1  LookupTableObject=''  BreakpointsForDimension1=SOC_BP  BreakpointsForDimension2=Temperature_BP  Table=Em  InterpMethod=Cubic spline  ExtrapMethod=Clip  UseLastTableValue=on  InternalRulePriority=Speed  RndMeth=Simplest  InputSameDT=on
  Em2 : Lookup_n-D  NumberOfTableDimensions=1  LookupTableObject=''  BreakpointsForDimension1=SOC_BP  BreakpointsForDimension2=Temperature_BP  Table=Em*Ns  InterpMethod=Cubic spline  ExtrapMethod=Clip  UseLastTableValue=on  InternalRulePriority=Speed  RndMeth=Simplest  InputSameDT=on
  Product : Product
  Ramp : simulink/Sources/Ramp  Commented=on  slope=-0.5  start=0  InitialOutput=1
  Scope1 : Scope
  Scope2 : Scope  Commented=on
  Subsystem : Subsystem
  Subsystem1 : Subsystem
  Vbatt : Outport
  Ploss : Outport  Port=2
  SOC : Outport  Port=3
  wires:
  Constant1/1 -> Product/1
  Constant2/1 -> Product/2, Subsystem/3(CapNom)
  Product/1 -> Subsystem/2(CapIni)
  Constant4/1 -> Subsystem1/2(Rseries)
  Ibatt/1 -> Subsystem1/3(Ibatt), Subsystem/1(I)
  Em2/1 -> Scope1/1, Subsystem1/1(Em)
  Subsystem1/1(Vbatt) -> Vbatt/1
  Subsystem/1(SOC) -> Em2/1, SOC/1
  Subsystem1/2(Ploss) -> Ploss/1
  Em1/1 -> Scope2/1
  Ramp/1 -> Em1/1

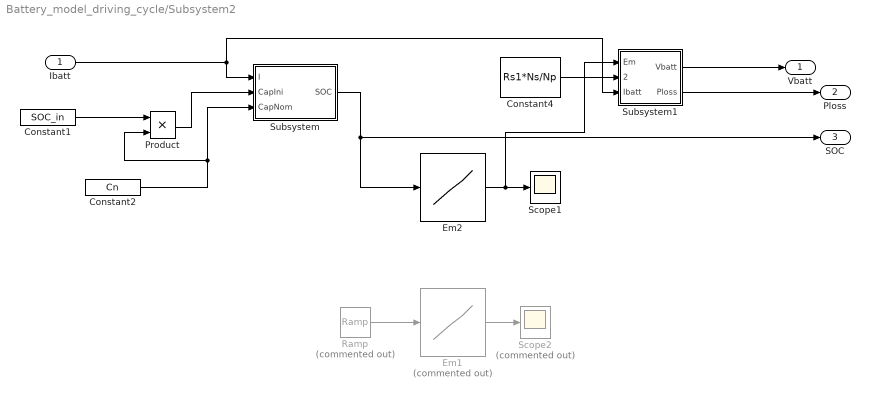
== system Battery_model_driving_cycle/Subsystem2 ==
  Ibatt : Inport
  Constant1 : Constant  Value=SOC_in  SampleTime=-1
  Constant2 : Constant  Value=Cn  SampleTime=-1
  Constant4 : Constant  Value=Rs1*Ns/Np  SampleTime=-1
  Em1 : Lookup_n-D  Commented=on  NumberOfTableDimensions=1  LookupTableObject=''  BreakpointsForDimension1=SOC_BP  BreakpointsForDimension2=Temperature_BP  Table=Em  InterpMethod=Cubic spline  ExtrapMethod=Clip  UseLastTableValue=on  InternalRulePriority=Speed  RndMeth=Simplest  InputSameDT=on
  Em2 : Lookup_n-D  NumberOfTableDimensions=1  LookupTableObject=''  BreakpointsForDimension1=SOC_BP  BreakpointsForDimension2=Temperature_BP  Table=Em*Ns  InterpMethod=Cubic spline  ExtrapMethod=Clip  UseLastTableValue=on  InternalRulePriority=Speed  RndMeth=Simplest  InputSameDT=on
  Product : Product
  Ramp : simulink/Sources/Ramp  Commented=on  slope=-0.5  start=0  InitialOutput=1
  Scope1 : Scope
  Scope2 : Scope  Commented=on
  Subsystem : Subsystem
  Subsystem1 : Subsystem
  Vbatt : Outport
  Ploss : Outport  Port=2
  SOC : Outport  Port=3
  wires:
  Ramp/1 -> Em1/1
  Em1/1 -> Scope2/1
  Subsystem1/2(Ploss) -> Ploss/1
  Subsystem/1(SOC) -> SOC/1, Em2/1
  Subsystem1/1(Vbatt) -> Vbatt/1
  Em2/1 -> Subsystem1/1(Em), Scope1/1
  Ibatt/1 -> Subsystem/1(I), Subsystem1/3(Ibatt)
  Constant4/1 -> Subsystem1/2(Rseries)
  Product/1 -> Subsystem/2(CapIni)
  Constant2/1 -> Subsystem/3(CapNom), Product/2
  Constant1/1 -> Product/1

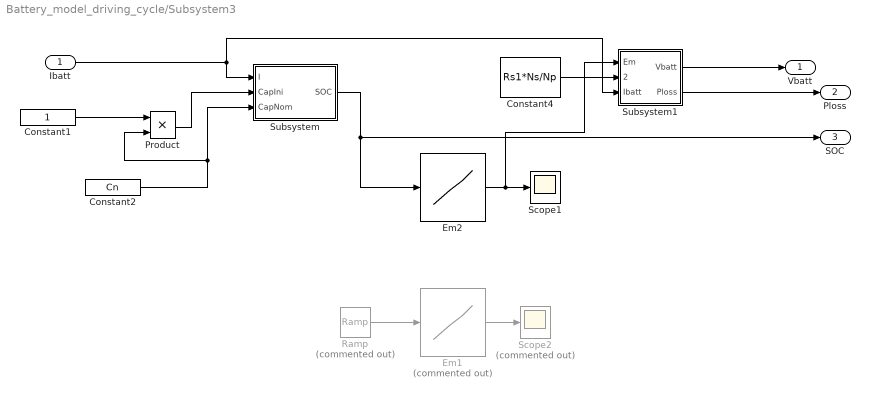
== system Battery_model_driving_cycle/Subsystem3 ==
  Ibatt : Inport
  Constant1 : Constant  SampleTime=-1
  Constant2 : Constant  Value=Cn  SampleTime=-1
  Constant4 : Constant  Value=Rs1*Ns/Np  SampleTime=-1
  Em1 : Lookup_n-D  Commented=on  NumberOfTableDimensions=1  LookupTableObject=''  BreakpointsForDimension1=SOC_BP  BreakpointsForDimension2=Temperature_BP  Table=Em  InterpMethod=Cubic spline  ExtrapMethod=Clip  UseLastTableValue=on  InternalRulePriority=Speed  RndMeth=Simplest  InputSameDT=on
  Em2 : Lookup_n-D  NumberOfTableDimensions=1  LookupTableObject=''  BreakpointsForDimension1=SOC_BP  BreakpointsForDimension2=Temperature_BP  Table=Em*Ns  InterpMethod=Cubic spline  ExtrapMethod=Clip  UseLastTableValue=on  InternalRulePriority=Speed  RndMeth=Simplest  InputSameDT=on
  Product : Product
  Ramp : simulink/Sources/Ramp  Commented=on  slope=-0.5  start=0  InitialOutput=1
  Scope1 : Scope
  Scope2 : Scope  Commented=on
  Subsystem : Subsystem
  Subsystem1 : Subsystem
  Vbatt : Outport
  Ploss : Outport  Port=2
  SOC : Outport  Port=3
  wires:
  Constant1/1 -> Product/1
  Constant2/1 -> Product/2, Subsystem/3(CapNom)
  Product/1 -> Subsystem/2(CapIni)
  Constant4/1 -> Subsystem1/2(Rseries)
  Ibatt/1 -> Subsystem1/3(Ibatt), Subsystem/1(I)
  Em2/1 -> Scope1/1, Subsystem1/1(Em)
  Subsystem1/1(Vbatt) -> Vbatt/1
  Subsystem/1(SOC) -> Em2/1, SOC/1
  Subsystem1/2(Ploss) -> Ploss/1
  Em1/1 -> Scope2/1
  Ramp/1 -> Em1/1

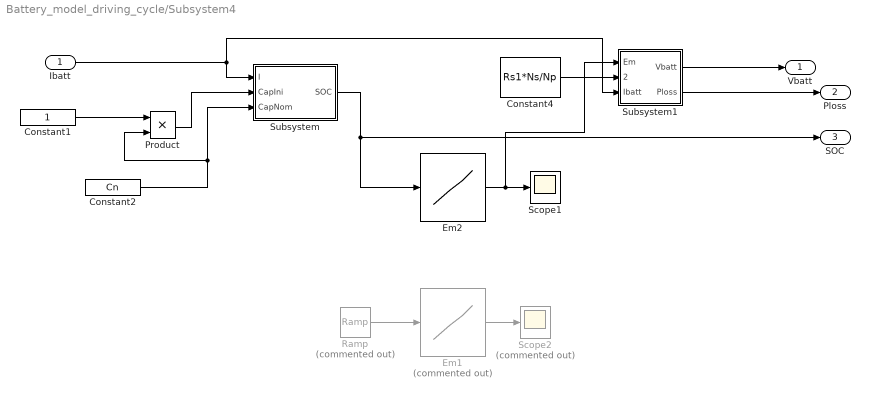
== system Battery_model_driving_cycle/Subsystem4 ==
  Ibatt : Inport
  Constant1 : Constant  SampleTime=-1
  Constant2 : Constant  Value=Cn  SampleTime=-1
  Constant4 : Constant  Value=Rs1*Ns/Np  SampleTime=-1
  Em1 : Lookup_n-D  Commented=on  NumberOfTableDimensions=1  LookupTableObject=''  BreakpointsForDimension1=SOC_BP  BreakpointsForDimension2=Temperature_BP  Table=Em  InterpMethod=Cubic spline  ExtrapMethod=Clip  UseLastTableValue=on  InternalRulePriority=Speed  RndMeth=Simplest  InputSameDT=on
  Em2 : Lookup_n-D  NumberOfTableDimensions=1  LookupTableObject=''  BreakpointsForDimension1=SOC_BP  BreakpointsForDimension2=Temperature_BP  Table=Em*Ns  InterpMethod=Cubic spline  ExtrapMethod=Clip  UseLastTableValue=on  InternalRulePriority=Speed  RndMeth=Simplest  InputSameDT=on
  Product : Product
  Ramp : simulink/Sources/Ramp  Commented=on  slope=-0.5  start=0  InitialOutput=1
  Scope1 : Scope
  Scope2 : Scope  Commented=on
  Subsystem : Subsystem
  Subsystem1 : Subsystem
  Vbatt : Outport
  Ploss : Outport  Port=2
  SOC : Outport  Port=3
  wires:
  Ramp/1 -> Em1/1
  Em1/1 -> Scope2/1
  Subsystem1/2(Ploss) -> Ploss/1
  Subsystem/1(SOC) -> SOC/1, Em2/1
  Subsystem1/1(Vbatt) -> Vbatt/1
  Em2/1 -> Subsystem1/1(Em), Scope1/1
  Ibatt/1 -> Subsystem/1(I), Subsystem1/3(Ibatt)
  Constant4/1 -> Subsystem1/2(Rseries)
  Product/1 -> Subsystem/2(CapIni)
  Constant2/1 -> Subsystem/3(CapNom), Product/2
  Constant1/1 -> Product/1

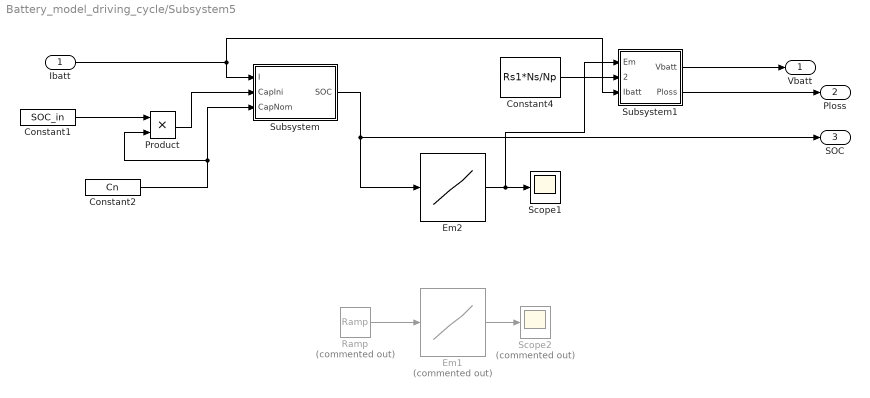
== system Battery_model_driving_cycle/Subsystem5 ==
  Ibatt : Inport
  Constant1 : Constant  Value=SOC_in  SampleTime=-1
  Constant2 : Constant  Value=Cn  SampleTime=-1
  Constant4 : Constant  Value=Rs1*Ns/Np  SampleTime=-1
  Em1 : Lookup_n-D  Commented=on  NumberOfTableDimensions=1  LookupTableObject=''  BreakpointsForDimension1=SOC_BP  BreakpointsForDimension2=Temperature_BP  Table=Em  InterpMethod=Cubic spline  ExtrapMethod=Clip  UseLastTableValue=on  InternalRulePriority=Speed  RndMeth=Simplest  InputSameDT=on
  Em2 : Lookup_n-D  NumberOfTableDimensions=1  LookupTableObject=''  BreakpointsForDimension1=SOC_BP  BreakpointsForDimension2=Temperature_BP  Table=Em*Ns  InterpMethod=Cubic spline  ExtrapMethod=Clip  UseLastTableValue=on  InternalRulePriority=Speed  RndMeth=Simplest  InputSameDT=on
  Product : Product
  Ramp : simulink/Sources/Ramp  Commented=on  slope=-0.5  start=0  InitialOutput=1
  Scope1 : Scope
  Scope2 : Scope  Commented=on
  Subsystem : Subsystem
  Subsystem1 : Subsystem
  Vbatt : Outport
  Ploss : Outport  Port=2
  SOC : Outport  Port=3
  wires:
  Constant1/1 -> Product/1
  Constant2/1 -> Product/2, Subsystem/3(CapNom)
  Product/1 -> Subsystem/2(CapIni)
  Constant4/1 -> Subsystem1/2(Rseries)
  Ibatt/1 -> Subsystem1/3(Ibatt), Subsystem/1(I)
  Em2/1 -> Scope1/1, Subsystem1/1(Em)
  Subsystem1/1(Vbatt) -> Vbatt/1
  Subsystem/1(SOC) -> Em2/1, SOC/1
  Subsystem1/2(Ploss) -> Ploss/1
  Em1/1 -> Scope2/1
  Ramp/1 -> Em1/1

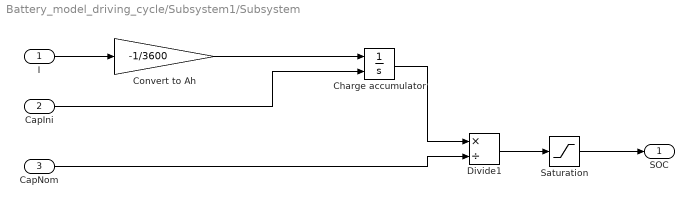
== system Battery_model_driving_cycle/Subsystem1/Subsystem ==
  I : Inport
  CapIni : Inport  Port=2
  CapNom : Inport  Port=3
  Charge accumulator : Integrator  InitialConditionSource=external  InitialCondition=Q_init*3600  LowerSaturationLimit=0
  Convert to Ah : Gain  Gain=-1/3600
  Divide1 : Product  Inputs=*/
  Saturation : Saturate  UpperLimit=1  LowerLimit=0
  SOC : Outport
  wires:
  I/1 -> Convert to Ah/1
  Saturation/1 -> SOC/1
  Charge accumulator/1 -> Divide1/1
  CapNom/1 -> Divide1/2
  CapIni/1 -> Charge accumulator/2
  Convert to Ah/1 -> Charge accumulator/1
  Divide1/1 -> Saturation/1

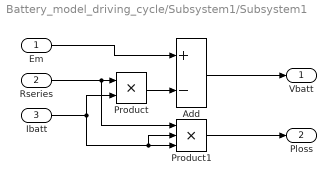
== system Battery_model_driving_cycle/Subsystem1/Subsystem1 ==
  Em : Inport
  Rseries : Inport  Port=2
  Ibatt : Inport  Port=3
  Add : Sum  Inputs=+-
  Product : Product
  Product1 : Product  Inputs=3
  Vbatt : Outport
  Ploss : Outport  Port=2
  wires:
  Ibatt/1 -> Product/2, Product1/3, Product1/2
  Product1/1 -> Ploss/1
  Rseries/1 -> Product/1, Product1/1
  Em/1 -> Add/1
  Add/1 -> Vbatt/1
  Product/1 -> Add/2

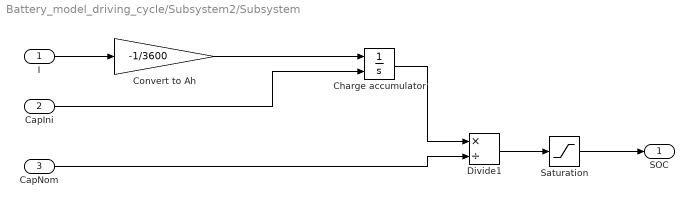
== system Battery_model_driving_cycle/Subsystem2/Subsystem ==
  I : Inport
  CapIni : Inport  Port=2
  CapNom : Inport  Port=3
  Charge accumulator : Integrator  InitialConditionSource=external  InitialCondition=Q_init*3600  LowerSaturationLimit=0
  Convert to Ah : Gain  Gain=-1/3600
  Divide1 : Product  Inputs=*/
  Saturation : Saturate  UpperLimit=1  LowerLimit=0
  SOC : Outport
  wires:
  Divide1/1 -> Saturation/1
  Convert to Ah/1 -> Charge accumulator/1
  CapIni/1 -> Charge accumulator/2
  CapNom/1 -> Divide1/2
  Charge accumulator/1 -> Divide1/1
  Saturation/1 -> SOC/1
  I/1 -> Convert to Ah/1

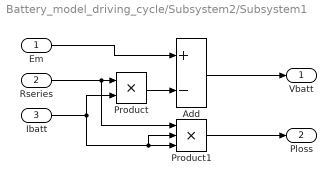
== system Battery_model_driving_cycle/Subsystem2/Subsystem1 ==
  Em : Inport
  Rseries : Inport  Port=2
  Ibatt : Inport  Port=3
  Add : Sum  Inputs=+-
  Product : Product
  Product1 : Product  Inputs=3
  Vbatt : Outport
  Ploss : Outport  Port=2
  wires:
  Product/1 -> Add/2
  Add/1 -> Vbatt/1
  Em/1 -> Add/1
  Rseries/1 -> Product1/1, Product/1
  Product1/1 -> Ploss/1
  Ibatt/1 -> Product1/2, Product1/3, Product/2

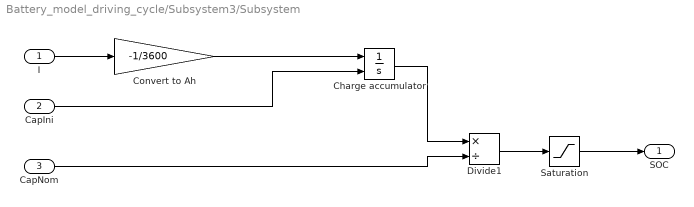
== system Battery_model_driving_cycle/Subsystem3/Subsystem ==
  I : Inport
  CapIni : Inport  Port=2
  CapNom : Inport  Port=3
  Charge accumulator : Integrator  InitialConditionSource=external  InitialCondition=Q_init*3600  LowerSaturationLimit=0
  Convert to Ah : Gain  Gain=-1/3600
  Divide1 : Product  Inputs=*/
  Saturation : Saturate  UpperLimit=1  LowerLimit=0
  SOC : Outport
  wires:
  I/1 -> Convert to Ah/1
  Saturation/1 -> SOC/1
  Charge accumulator/1 -> Divide1/1
  CapNom/1 -> Divide1/2
  CapIni/1 -> Charge accumulator/2
  Convert to Ah/1 -> Charge accumulator/1
  Divide1/1 -> Saturation/1

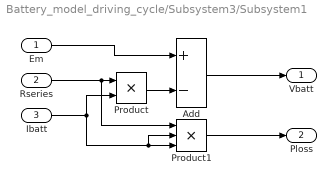
== system Battery_model_driving_cycle/Subsystem3/Subsystem1 ==
  Em : Inport
  Rseries : Inport  Port=2
  Ibatt : Inport  Port=3
  Add : Sum  Inputs=+-
  Product : Product
  Product1 : Product  Inputs=3
  Vbatt : Outport
  Ploss : Outport  Port=2
  wires:
  Ibatt/1 -> Product/2, Product1/3, Product1/2
  Product1/1 -> Ploss/1
  Rseries/1 -> Product/1, Product1/1
  Em/1 -> Add/1
  Add/1 -> Vbatt/1
  Product/1 -> Add/2

== system Battery_model_driving_cycle/Subsystem4/Subsystem ==
  I : Inport
  CapIni : Inport  Port=2
  CapNom : Inport  Port=3
  Charge accumulator : Integrator  InitialConditionSource=external  InitialCondition=Q_init*3600  LowerSaturationLimit=0
  Convert to Ah : Gain  Gain=-1/3600
  Divide1 : Product  Inputs=*/
  Saturation : Saturate  UpperLimit=1  LowerLimit=0
  SOC : Outport
  wires:
  Divide1/1 -> Saturation/1
  Convert to Ah/1 -> Charge accumulator/1
  CapIni/1 -> Charge accumulator/2
  CapNom/1 -> Divide1/2
  Charge accumulator/1 -> Divide1/1
  Saturation/1 -> SOC/1
  I/1 -> Convert to Ah/1

== system Battery_model_driving_cycle/Subsystem4/Subsystem1 ==
  Em : Inport
  Rseries : Inport  Port=2
  Ibatt : Inport  Port=3
  Add : Sum  Inputs=+-
  Product : Product
  Product1 : Product  Inputs=3
  Vbatt : Outport
  Ploss : Outport  Port=2
  wires:
  Product/1 -> Add/2
  Add/1 -> Vbatt/1
  Em/1 -> Add/1
  Rseries/1 -> Product1/1, Product/1
  Product1/1 -> Ploss/1
  Ibatt/1 -> Product1/2, Product1/3, Product/2

== system Battery_model_driving_cycle/Subsystem5/Subsystem ==
  I : Inport
  CapIni : Inport  Port=2
  CapNom : Inport  Port=3
  Charge accumulator : Integrator  InitialConditionSource=external  InitialCondition=Q_init*3600  LowerSaturationLimit=0
  Convert to Ah : Gain  Gain=-1/3600
  Divide1 : Product  Inputs=*/
  Saturation : Saturate  UpperLimit=1  LowerLimit=0
  SOC : Outport
  wires:
  I/1 -> Convert to Ah/1
  Saturation/1 -> SOC/1
  Charge accumulator/1 -> Divide1/1
  CapNom/1 -> Divide1/2
  CapIni/1 -> Charge accumulator/2
  Convert to Ah/1 -> Charge accumulator/1
  Divide1/1 -> Saturation/1

== system Battery_model_driving_cycle/Subsystem5/Subsystem1 ==
  Em : Inport
  Rseries : Inport  Port=2
  Ibatt : Inport  Port=3
  Add : Sum  Inputs=+-
  Product : Product
  Product1 : Product  Inputs=3
  Vbatt : Outport
  Ploss : Outport  Port=2
  wires:
  Ibatt/1 -> Product/2, Product1/3, Product1/2
  Product1/1 -> Ploss/1
  Rseries/1 -> Product/1, Product1/1
  Em/1 -> Add/1
  Add/1 -> Vbatt/1
  Product/1 -> Add/2
